simulink model "LaneTracking"  (R2023b)
settings: Solver=ode4  StartTime=0.0  StopTime=Te  FixedStep=Ts  RelTol=1e-3
undefined symbols (not defined in the file): driving, egoCarID, targetSpeed, Ts
libraries: drivingscenarioandsensors x7, slpidlib x2, robotcorelib x2, sensorinslib x1
(part 1 of 3)
settings Model: NumberOfSteps=10  SnapshotBufferSize=1000  SnapshotInterval=100  Creator=Victor  LastModifiedBy=victor
settings SolverCC: ZeroCrossAlgorithm=Adaptive
settings DebuggingCC: IgnoredZcDiagnostic=none
settings RTWCC: Toolchain=MinGW64 | CMake/gmake (64-bit Windows)  BuildConfiguration=Release

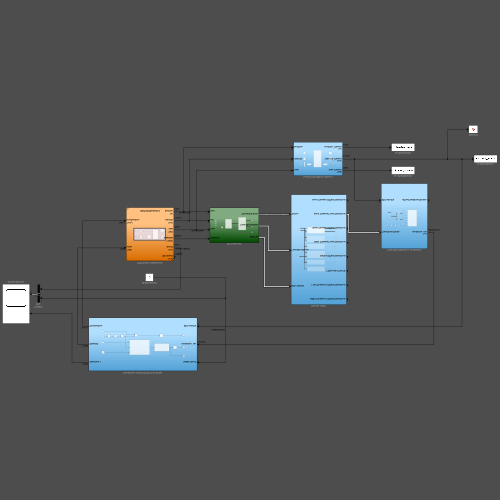
[thumbnail: Simulink's stored preview of the top-level diagram]
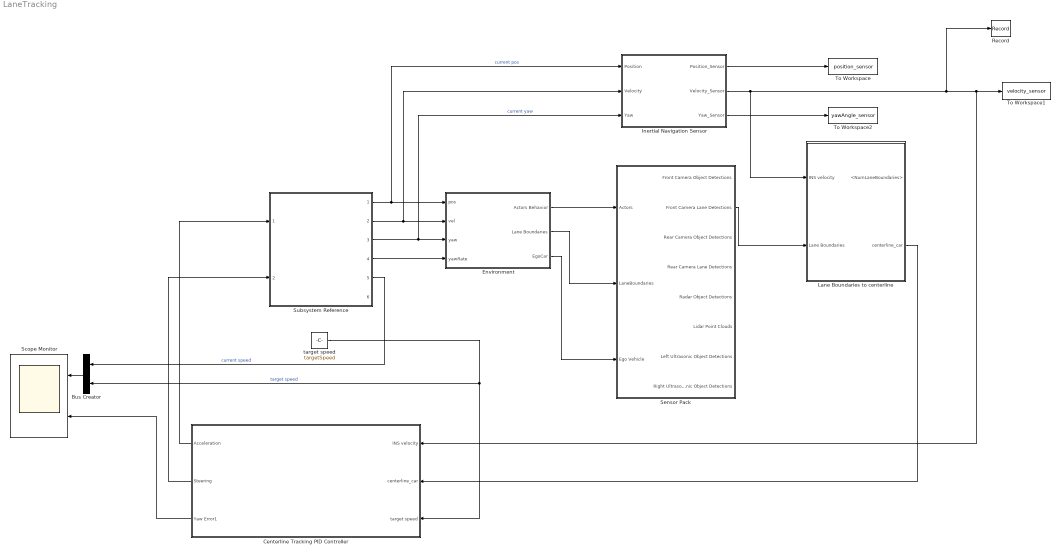
== system LaneTracking ==
  Bus Creator : BusCreator  Inputs=2
  Centerline Tracking PID Controller : Subsystem
  Environment : Subsystem
  Inertial Navigation Sensor : Subsystem
  Lane Boundaries to centerline : Subsystem
  Record : Record  FileSettingsInternal="{\"entries\":[{\"content\":{\"excelSettings\":{\"content\":{},\"type\":\"Streamout.ExcelSettings\"}},\"type\":\"Streamout.FileSettingStorage\",\"uuid\":\"\"}],\"packageUris\":[\"http:\\/\\/schema.mathworks.com\\/mf0\\/streamout_blocks\\/R2020a\"],\"version\":\"1.0\"}"  Layout=[2 1]  SignalsInternal="{\"entries\":[{\"content\":{\"signals\":[{\"content\":{\"blockPath\":[],\"dimensions\":[2],\"domain\":\"\",\"hasChildren\":true,\"lineColor\":\"#0072bd\",\"port\":1,\"sid\":[\"\"],\"signalID\":63381,\"signalName\":\"Inertial Navigation Sensor:2\"},\"type\":\"RecordBlkView.Signal\",\"uuid\":\"\"},{\"content\":{\"blockPath\":[],\"channel\":[1],\"dimensions\":[2],\"domain\":\"\",\"lineColor\":\"#139fff\",\"parentID\":63381,\"plots\":[1],\"port\":1,\"sid\":[\"\"],\"signalID\":63382,\"signalName\":\"Inertial Navigation Sensor:2\"},\"type\":\"RecordBlkView.Signal\",\"uuid\":\"\"},{\"content\":{\"blockPath\":[],\"channel\":[2],\"dimensions\":[2],\"domain\":\"\",\"lineColor\":\"#a2142f\",\"parentID\":63381,\"plots\":[2],\"port\":1,\"sid\":[\"\"],\"signalID\":65349,\"signalName\":\"Inertial Navigation Sensor:2\"},\"type\":\"RecordBlkView.Signal\",\"uuid\":\"\"}]},\"type\":\"RecordBlkView.InputSignals\",\"uuid\":\"\"}],\"packageUris\":[\"http:\\/\\/schema.mathworks.com\\/mf0\\/streamout_blocks\\/R2020a\"],\"version\":\"1.0\"}"
  Scope Monitor : Scope  NumInputPorts=2
  Sensor Pack : Subsystem
  Subsystem Reference : Subsystem  ReferencedSubsystem=VehicleDynamics
  To Workspace : ToWorkspace  VariableName=position_sensor  SampleTime=-1
  To Workspace1 : ToWorkspace  VariableName=velocity_sensor  SampleTime=-1
  To Workspace2 : ToWorkspace  VariableName=yawAngle_sensor  SampleTime=-1
  target speed : Constant  Value=targetSpeed
  wires:
  Subsystem Reference/1 -> Environment/1(pos), Inertial Navigation Sensor/1(Position)  "current pos"
  Subsystem Reference/2 -> Inertial Navigation Sensor/2(Velocity), Environment/2(vel)
  Subsystem Reference/3 -> Inertial Navigation Sensor/3(Yaw), Environment/3(yaw)  "current yaw"
  Subsystem Reference/4 -> Environment/4(yawRate)
  Environment/1(Actors Behavior) -> Sensor Pack/1(Actors)
  Environment/2(Lane Boundaries) -> Sensor Pack/2(LaneBoundaries)
  Environment/3(EgoCar) -> Sensor Pack/3(Ego Vehicle)
  Sensor Pack/2(Front Camera Lane Detections) -> Lane Boundaries to centerline/2(Lane Boundaries)
  target speed/1 -> Centerline Tracking PID Controller/3(target speed), Bus Creator/2  "target speed"
  Subsystem Reference/5 -> Bus Creator/1  "current speed"
  Bus Creator/1 -> Scope Monitor/1
  Inertial Navigation Sensor/1(Position_Sensor) -> To Workspace/1
  Inertial Navigation Sensor/2(Velocity_Sensor) -> Lane Boundaries to centerline/1(INS velocity), Record/1, Centerline Tracking PID Controller/1(INS velocity), To Workspace1/1
  Inertial Navigation Sensor/3(Yaw_Sensor) -> To Workspace2/1
  Lane Boundaries to centerline/2(centerline_car) -> Centerline Tracking PID Controller/2(centerline_car)
  Centerline Tracking PID Controller/1(Acceleration) -> Subsystem Reference/1
  Centerline Tracking PID Controller/2(Steering) -> Subsystem Reference/2
  Centerline Tracking PID Controller/3(Yaw Error1) -> Scope Monitor/2

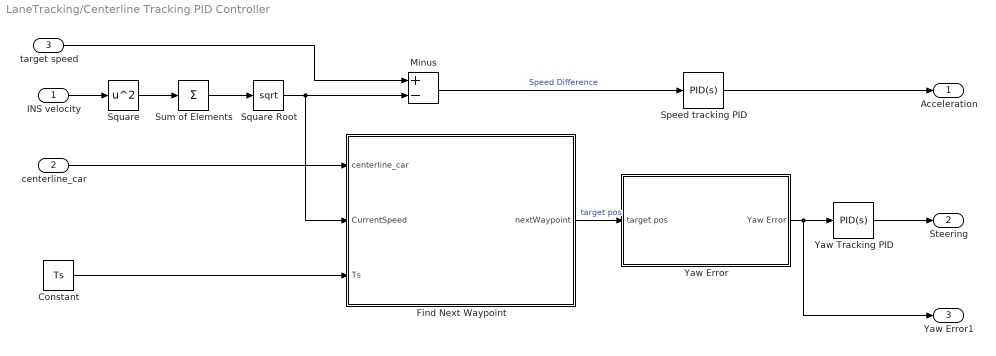
== system LaneTracking/Centerline Tracking PID Controller ==
  INS velocity : Inport
  centerline_car : Inport  Port=2
  target speed : Inport  Port=3
  Constant : Constant  Value=Ts
  Find Next Waypoint : MATLAB Function  TreatAsAtomicUnit=on
  Minus : Sum  Inputs=+-
  Speed tracking PID : slpidlib/PID Controller  Controller=PID  Form=Parallel  TimeDomain=Continuous-time  UseExternalTs=off  SampleTime=-1  IntegratorMethod=Forward Euler  FilterMethod=Forward Euler  ControllerParametersSource=internal  P=9E-1  I=0  UseKiTs=off  D=1e-3  N=100  UseFilter=on  TunerSelectOption=Transfer Function Based (PID Tuner App)  InitialConditionSource=internal  InitialConditionForIntegrator=0  InitialConditionForFilter=0  DifferentiatorICPrevScaledInput=0  ExternalReset=none  TrackingMode=off  Kt=1  LimitOutput=off  SatLimitsSource=internal  UpperSaturationLimit=inf  LowerSaturationLimit=-inf  LinearizeAsGain=on  AntiWindupMode=none  Kb=1  LimitIntegrator=off  UpperIntegratorSaturationLimit=inf  LowerIntegratorSaturationLimit=-inf  POutMin=[]  POutMax=[]  IOutMin=[]  IOutMax=[]  DOutMin=[]  DOutMax=[]  NOutMin=[]  NOutMax=[]  SumOutMin=[]  SumOutMax=[]  SaturationOutMin=[]  SaturationOutMax=[]  PParamMin=[]  PParamMax=[]  IParamMin=[]  IParamMax=[]  DParamMin=[]  DParamMax=[]  NParamMin=[]  NParamMax=[]  KbParamMin=[]  KbParamMax=[]  KtParamMin=[]  KtParamMax=[]  KbOutMin=[]  KbOutMax=[]  KtOutMin=[]  KtOutMax=[]  IntegratorOutMin=[]  IntegratorOutMax=[]  FilterOutMin=[]  FilterOutMax=[]  SumI1OutMin=[]  SumI1OutMax=[]  SumI2OutMin=[]  SumI2OutMax=[]  SumI3OutMin=[]  SumI3OutMax=[]  SumI4OutMin=[]  SumI4OutMax=[]  SumDOutMin=[]  SumDOutMax=[]  DifferentiatorOutMin=[]  DifferentiatorOutMax=[]  FilterDiffOutCoefMin=[]  FilterDiffOutCoefMax=[]  ReciprocalOutMin=[]  ReciprocalOutMax=[]  SumDenOutMin=[]  SumDenOutMax=[]  SumNumOutMin=[]  SumNumOutMax=[]  DivideOutMin=[]  DivideOutMax=[]  UdiffTsProdOutMin=[]  UdiffTsProdOutMax=[]  NTsProdOutMin=[]  NTsProdOutMax=[]  UintegralTsProdOutMin=[]  UintegralTsProdOutMax=[]  UngainTsProdOutMin=[]  UngainTsProdOutMax=[]  ClampingZeroOutDataTypeStr=Inherit: Inherit via back propagation  ClampingZeroOutMin=[]  ClampingZeroOutMax=[]  FilterDenConstantOutDataTypeStr=Inherit: Inherit via back propagation  FilterDenConstantOutMin=[]  FilterDenConstantOutMax=[]  PCopyOutDataTypeStr=Inherit: Inherit via back propagation  PCopyOutMin=[]  PCopyOutMax=[]  NCopyOutDataTypeStr=Inherit: Inherit via back propagation  NCopyOutMin=[]  NCopyOutMax=[]  IntegratorContinuousStateAttributes=''  IntegratorStateMustResolveToSignalObject=off  IntegratorRTWStateStorageClass=Auto  FilterContinuousStateAttributes=''  FilterStateMustResolveToSignalObject=off  FilterRTWStateStorageClass=Auto  ParallelPVariant=InternalParameters  IdealPVariant=Disabled  IVariant=InternalParameters  DVariant=InternalParameters  IntegratorVariant=Continuous  SatVariant=Disabled  AWVariant=Passthrough  PCopyVariant=Disabled  TRVariant=Disabled  FdbkBlocksVariant=Forward  IdealPFdbkVariant=Disabled  SatFdbkVariant=Disabled  DerivativeFilterVariant=ContFilter  NVariant=InternalParameters  NCopyVariant=Disabled  FilterICVariant=InternalICsFilter  IntegratorICVariant=InternalICs  ExternalResetVariant=Disabled  TRSumVariant=Passthrough  SumFdbkVariant=Disabled  SumVariant=Sum_PID  TsampFilterVariant=InternalTs  TsampNgainVariant=Passthrough  TsampIntegralVariant=Disabled_SignalSpec  ExternalSaturationOutDataTypeStr=Inherit: Same as second input
  Square : Math  Operator=square
  Square Root : Sqrt
  Sum of Elements : Sum  Inputs=+
  Yaw Error : Subsystem
  Yaw Tracking PID : slpidlib/PID Controller  Controller=PID  Form=Parallel  TimeDomain=Continuous-time  UseExternalTs=off  SampleTime=-1  IntegratorMethod=Forward Euler  FilterMethod=Forward Euler  ControllerParametersSource=internal  P=3.5E-3  I=1.5E-3  UseKiTs=on  D=1.7E-3  N=100  UseFilter=on  TunerSelectOption=Transfer Function Based (PID Tuner App)  InitialConditionSource=internal  InitialConditionForIntegrator=0  InitialConditionForFilter=0  DifferentiatorICPrevScaledInput=0  ExternalReset=none  TrackingMode=off  Kt=1  LimitOutput=off  SatLimitsSource=internal  UpperSaturationLimit=inf  LowerSaturationLimit=-inf  LinearizeAsGain=on  AntiWindupMode=none  Kb=1  LimitIntegrator=off  UpperIntegratorSaturationLimit=inf  LowerIntegratorSaturationLimit=-inf  POutMin=[]  POutMax=[]  IOutMin=[]  IOutMax=[]  DOutMin=[]  DOutMax=[]  NOutMin=[]  NOutMax=[]  SumOutMin=[]  SumOutMax=[]  SaturationOutMin=[]  SaturationOutMax=[]  PParamMin=[]  PParamMax=[]  IParamMin=[]  IParamMax=[]  DParamMin=[]  DParamMax=[]  NParamMin=[]  NParamMax=[]  KbParamMin=[]  KbParamMax=[]  KtParamMin=[]  KtParamMax=[]  KbOutMin=[]  KbOutMax=[]  KtOutMin=[]  KtOutMax=[]  IntegratorOutMin=[]  IntegratorOutMax=[]  FilterOutMin=[]  FilterOutMax=[]  SumI1OutMin=[]  SumI1OutMax=[]  SumI2OutMin=[]  SumI2OutMax=[]  SumI3OutMin=[]  SumI3OutMax=[]  SumI4OutMin=[]  SumI4OutMax=[]  SumDOutMin=[]  SumDOutMax=[]  DifferentiatorOutMin=[]  DifferentiatorOutMax=[]  FilterDiffOutCoefMin=[]  FilterDiffOutCoefMax=[]  ReciprocalOutMin=[]  ReciprocalOutMax=[]  SumDenOutMin=[]  SumDenOutMax=[]  SumNumOutMin=[]  SumNumOutMax=[]  DivideOutMin=[]  DivideOutMax=[]  UdiffTsProdOutMin=[]  UdiffTsProdOutMax=[]  NTsProdOutMin=[]  NTsProdOutMax=[]  UintegralTsProdOutMin=[]  UintegralTsProdOutMax=[]  UngainTsProdOutMin=[]  UngainTsProdOutMax=[]  ClampingZeroOutDataTypeStr=Inherit: Inherit via back propagation  ClampingZeroOutMin=[]  ClampingZeroOutMax=[]  FilterDenConstantOutDataTypeStr=Inherit: Inherit via back propagation  FilterDenConstantOutMin=[]  FilterDenConstantOutMax=[]  PCopyOutDataTypeStr=Inherit: Inherit via back propagation  PCopyOutMin=[]  PCopyOutMax=[]  NCopyOutDataTypeStr=Inherit: Inherit via back propagation  NCopyOutMin=[]  NCopyOutMax=[]  IntegratorContinuousStateAttributes=''  IntegratorStateMustResolveToSignalObject=off  IntegratorRTWStateStorageClass=Auto  FilterContinuousStateAttributes=''  FilterStateMustResolveToSignalObject=off  FilterRTWStateStorageClass=Auto  ParallelPVariant=InternalParameters  IdealPVariant=Disabled  IVariant=InternalParameters  DVariant=InternalParameters  IntegratorVariant=Continuous  SatVariant=Disabled  AWVariant=Passthrough  PCopyVariant=Disabled  TRVariant=Disabled  FdbkBlocksVariant=Forward  IdealPFdbkVariant=Disabled  SatFdbkVariant=Disabled  DerivativeFilterVariant=ContFilter  NVariant=InternalParameters  NCopyVariant=Disabled  FilterICVariant=InternalICsFilter  IntegratorICVariant=InternalICs  ExternalResetVariant=Disabled  TRSumVariant=Passthrough  SumFdbkVariant=Disabled  SumVariant=Sum_PID  TsampFilterVariant=InternalTs  TsampNgainVariant=Passthrough  TsampIntegralVariant=Disabled_SignalSpec  ExternalSaturationOutDataTypeStr=Inherit: Same as second input
  Acceleration : Outport
  Steering : Outport  Port=2
  Yaw Error1 : Outport  Port=3
  wires:
  Yaw Tracking PID/1 -> Steering/1
  Minus/1 -> Speed tracking PID/1  "Speed Difference"
  Yaw Error/1(Yaw Error) -> Yaw Tracking PID/1, Yaw Error1/1
  Find Next Waypoint/1(nextWaypoint) -> Yaw Error/1(target pos)  "target pos"
  Constant/1 -> Find Next Waypoint/3(Ts)
  Speed tracking PID/1 -> Acceleration/1
  Square Root/1 -> Find Next Waypoint/2(CurrentSpeed), Minus/2
  centerline_car/1 -> Find Next Waypoint/1(centerline_car)
  INS velocity/1 -> Square/1
  Sum of Elements/1 -> Square Root/1
  Square/1 -> Sum of Elements/1
  target speed/1 -> Minus/1

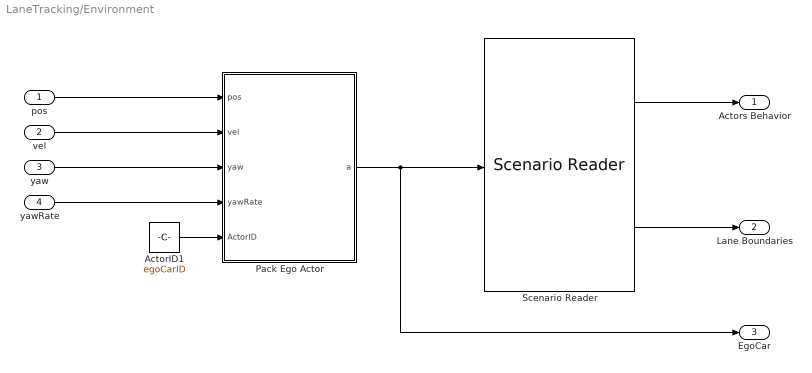
== system LaneTracking/Environment ==
  pos : Inport
  vel : Inport  Port=2
  yaw : Inport  Port=3
  yawRate : Inport  Port=4
  ActorID1 : Constant  Value=egoCarID
  Pack Ego Actor : MATLAB Function  TreatAsAtomicUnit=on
  Scenario Reader : drivingscenarioandsensors/Scenario Reader  ScenarioSource=From file  ScenarioFileName=Scenario_OneEgoCar.mat  ScenarioVariableName=scenario  OutputCoordinateSystem=Vehicle coordinates  EgoVehicleSource=Input port  EgoVehicleActorID=egoCarID  OrientVehiclesOnRoad=on  OutputEgoVehiclePose=off  OutputEgoVehicleState=off  SampleTime=Ts  LaneBoundaryOutput=Ego vehicle lane boundaries  LaneBoundaryDistance=0:0.5:60  LaneBoundaryLocation=Inner edge of lane markings  BusNameSource=Auto  BusName=BusActorsActors  BusNumActorsSource=Scenario  BusNumActors=100  BusName2Source=Auto  BusName2=BusLaneBoundaries  BusNumLaneBoundariesSource=Scenario  BusNumLaneBoundaries=10  BusName3Source=Auto  BusName3=BusEgoActor  BusName4Source=Auto  BusName4=BusEgoState  ShowCoordinateLabels=on  SimulateUsing=Code generation
  Actors Behavior : Outport
  Lane Boundaries : Outport  Port=2
  EgoCar : Outport  Port=3
  wires:
  pos/1 -> Pack Ego Actor/1(pos)
  Pack Ego Actor/1(a) -> Scenario Reader/1, EgoCar/1
  ActorID1/1 -> Pack Ego Actor/5(ActorID)
  Scenario Reader/1 -> Actors Behavior/1
  vel/1 -> Pack Ego Actor/2(vel)
  yaw/1 -> Pack Ego Actor/3(yaw)
  yawRate/1 -> Pack Ego Actor/4(yawRate)
  Scenario Reader/2 -> Lane Boundaries/1

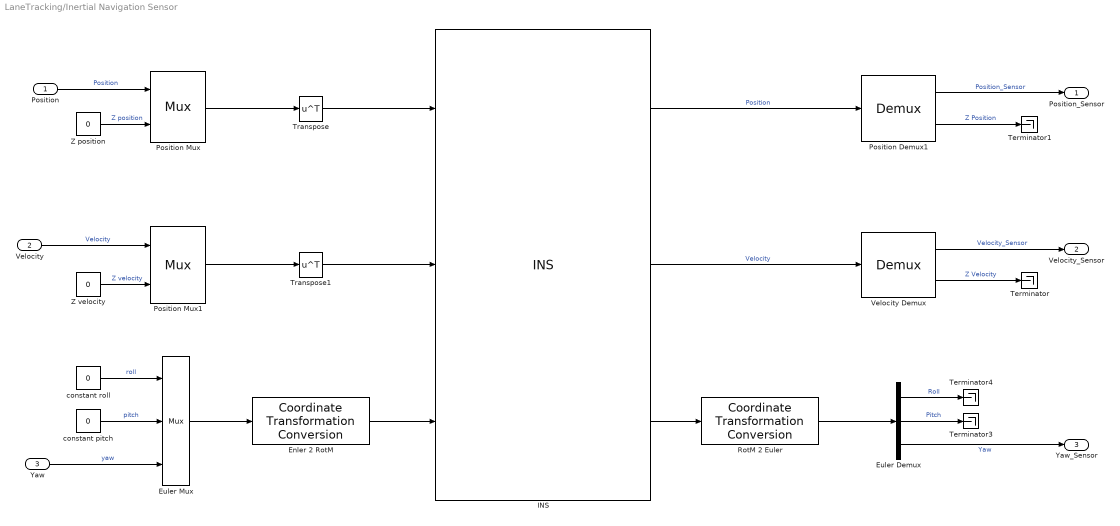
== system LaneTracking/Inertial Navigation Sensor ==
  Position : Inport
  Velocity : Inport  Port=2
  Yaw : Inport  Port=3
  Enler 2 RotM : robotcorelib/Coordinate Transformation Conversion  InputRepresentation=Euler Angles  InputEulerSequence=XYZ  ShowTrVecInputPort=on  OutputRepresentation=Rotation Matrix  OutputEulerSequence=XYZ  ShowTrVecOutputPort=on  SimulateUsing=Code generation
      settings: LibrarySourceBlock=uavutilslib/Coordinate Transformation Conversion
  Euler Demux : Demux  Outputs=3
      settings: DisplayOption=none
  Euler Mux : Mux  Inputs=3
      settings: DisplayOption=signals
  INS : sensorinslib/INS  MountingLocation=[0 0 0]  RollAccuracy=angleAccuraccy  PitchAccuracy=angleAccuraccy  YawAccuracy=angleAccuraccy  PositionAccuracy=positionAccuracy  VelocityAccuracy=velocityAccuracy  UseAccelAndAngVel=off  AccelerationAccuracy=0  AngularVelocityAccuracy=0  TimeInput=off  PositionErrorFactor=[0 0 0]  SeedDouble=32  SimulateUsing=Code generation
      settings: LibrarySourceBlock=drivingscenarioandsensors/INS
  Position Demux1 : Demux  Outputs=2
      settings: DisplayOption=none
  Position Mux : Mux  Inputs=2
      settings: DisplayOption=signals
  Position Mux1 : Mux  Inputs=2
      settings: DisplayOption=signals
  RotM 2 Euler : robotcorelib/Coordinate Transformation Conversion  InputRepresentation=Rotation Matrix  InputEulerSequence=XYZ  ShowTrVecInputPort=on  OutputRepresentation=Euler Angles  OutputEulerSequence=XYZ  ShowTrVecOutputPort=on  SimulateUsing=Code generation
      settings: LibrarySourceBlock=uavutilslib/Coordinate Transformation Conversion
  Terminator{,1,3..4} (4 alike) : Terminator
  Transpose : Math  Operator=transpose
  Transpose1 : Math  Operator=transpose
  Velocity Demux : Demux  Outputs=2
      settings: DisplayOption=none
  Z position : Constant  Value=0
  Z velocity : Constant  Value=0
  constant pitch : Constant  Value=0
  constant roll : Constant  Value=0
  Position_Sensor : Outport  Unit=m  PortDimensions=2
  Velocity_Sensor : Outport  Port=2  Unit=m/s  PortDimensions=2
  Yaw_Sensor : Outport  Port=3  Unit=deg
  wires:
  Enler 2 RotM/1 -> INS/3
  Euler Demux/1 -> Terminator4/1  "Roll"
  Euler Mux/1 -> Enler 2 RotM/1
  RotM 2 Euler/1 -> Euler Demux/1
  Euler Demux/3 -> Yaw_Sensor/1  "Yaw"
  INS/3 -> RotM 2 Euler/1
  Euler Demux/2 -> Terminator3/1  "Pitch"
  constant roll/1 -> Euler Mux/1  "roll"
  constant pitch/1 -> Euler Mux/2  "pitch"
  Yaw/1 -> Euler Mux/3  "yaw"
  Position/1 -> Position Mux/1  "Position"
  Z position/1 -> Position Mux/2  "Z position"
  Z velocity/1 -> Position Mux1/2  "Z velocity"
  Velocity/1 -> Position Mux1/1  "Velocity"
  Position Mux/1 -> Transpose/1
  Transpose/1 -> INS/1
  Position Mux1/1 -> Transpose1/1
  Transpose1/1 -> INS/2
  INS/2 -> Velocity Demux/1  "Velocity"
  Velocity Demux/1 -> Velocity_Sensor/1  "Velocity_Sensor"
  Velocity Demux/2 -> Terminator/1  "Z Velocity"
  Position Demux1/1 -> Position_Sensor/1  "Position_Sensor"
  Position Demux1/2 -> Terminator1/1  "Z Position"
  INS/1 -> Position Demux1/1  "Position"

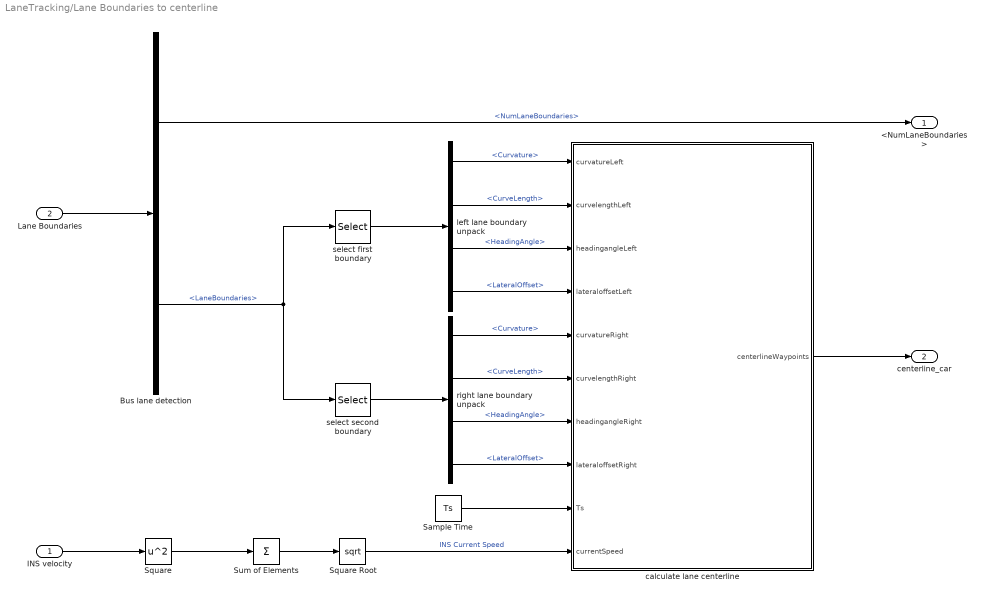
== system LaneTracking/Lane Boundaries to centerline ==
  INS velocity : Inport
  Lane Boundaries : Inport  Port=2
  Bus lane detection : BusSelector  OutputSignals=NumLaneBoundaries,LaneBoundaries
  Sample Time : Constant  Value=Ts
  Square : Math  Operator=square
  Square Root : Sqrt
  Sum of Elements : Sum  Inputs=+
  "calculate lane centerline " : MATLAB Function  TreatAsAtomicUnit=on
  left lane boundary unpack : BusSelector  OutputSignals=Curvature,CurveLength,HeadingAngle,LateralOffset
  right lane boundary unpack : BusSelector  OutputSignals=Curvature,CurveLength,HeadingAngle,LateralOffset
  select first boundary : Selector  InputPortWidth=4  IndexOptions=Index vector (dialog)  Indices=[1]  OutputSizes=1
  select second boundary : Selector  InputPortWidth=4  IndexOptions=Index vector (dialog)  Indices=[2]  OutputSizes=1
  <NumLaneBoundaries> : Outport
  centerline_car : Outport  Port=2  Unit=m
  wires:
  right lane boundary unpack/3 -> "calculate lane centerline "/7(headingangleRight)  "<HeadingAngle>"
  select first boundary/1 -> left lane boundary unpack/1
  left lane boundary unpack/4 -> "calculate lane centerline "/4(lateraloffsetLeft)  "<LateralOffset>"
  left lane boundary unpack/2 -> "calculate lane centerline "/2(curvelengthLeft)  "<CurveLength>"
  Bus lane detection/2 -> select second boundary/1, select first boundary/1  "<LaneBoundaries>"
  right lane boundary unpack/1 -> "calculate lane centerline "/5(curvatureRight)  "<Curvature>"
  right lane boundary unpack/4 -> "calculate lane centerline "/8(lateraloffsetRight)  "<LateralOffset>"
  select second boundary/1 -> right lane boundary unpack/1
  right lane boundary unpack/2 -> "calculate lane centerline "/6(curvelengthRight)  "<CurveLength>"
  left lane boundary unpack/3 -> "calculate lane centerline "/3(headingangleLeft)  "<HeadingAngle>"
  left lane boundary unpack/1 -> "calculate lane centerline "/1(curvatureLeft)  "<Curvature>"
  Bus lane detection/1 -> <NumLaneBoundaries>/1  "<NumLaneBoundaries>"
  Lane Boundaries/1 -> Bus lane detection/1
  "calculate lane centerline "/1(centerlineWaypoints) -> centerline_car/1
  Sample Time/1 -> "calculate lane centerline "/9(Ts)
  INS velocity/1 -> Square/1
  Square/1 -> Sum of Elements/1
  Square Root/1 -> "calculate lane centerline "/10(currentSpeed)  "INS Current Speed"
  Sum of Elements/1 -> Square Root/1
